simulink model "montecar"  (Simulink 4.00)
settings: Solver=VariableStepDiscrete  SolverMode=SingleTasking  StartTime=0.0  StopTime=10  FixedStep=1  MaxStep=1  RelTol=1e-3  AbsTol=1e-6
PreLoadFcn:
  | monteset
StopFcn:
  | monteplo
undefined symbols (not defined in the file or in its folder): fcost, invest, k, mshare, msize, pow, rate, ucost, uprice
CloseFcn:
  | close(findobj('name','Business Model Graph'))
settings Model: RequirementInfo=9  Creator=pseca  LastModifiedBy=eyarrow  SaveTime=off  SaveOutput=off  LimitDataPoints=off  RTWTemplateMakefile=grt_vc.tmf  BlockReductionOpt=off

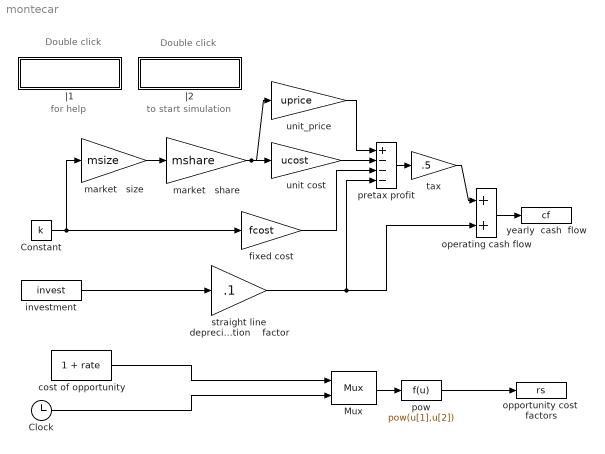
== system montecar ==
  note: Double click
  note: for help
  note: Double click
  note: to start simulation
  " straight line depreciation    factor" : Gain  Gain=.1  Multiplication=Element-wise(K.*u)  SaturateOnIntegerOverflow=on
  Clock : Clock
      settings: Decimation=10
  Constant : Constant  Value=k
  Mux : Mux  Inputs=2
      settings: DisplayOption=none
  "cost of opportunity " : Constant  Value=1 + rate
  fixed cost : Gain  Gain=fcost  Multiplication=Element-wise(K.*u)  SaturateOnIntegerOverflow=on
  investment : Constant  Value=invest
  market   share : Gain  Gain=mshare  Multiplication=Element-wise(K.*u)  SaturateOnIntegerOverflow=on
  market   size : Gain  Gain=msize  Multiplication=Element-wise(K.*u)  SaturateOnIntegerOverflow=on
  operating cash flow : Sum  Inputs=++  SaturateOnIntegerOverflow=on
  opportunity cost  factors : ToWorkspace  VariableName=rs  SampleTime=0  SaveFormat=Array
      settings: MaxDataPoints=10
  pow : Fcn  Expr=pow(u[1],u[2])
  pretax profit : Sum  Inputs=+---  SaturateOnIntegerOverflow=on
  tax : Gain  Gain=.5  Multiplication=Element-wise(K.*u)  SaturateOnIntegerOverflow=on
  unit cost : Gain  Gain=ucost  Multiplication=Element-wise(K.*u)  SaturateOnIntegerOverflow=on
  unit_price : Gain  Gain=uprice  Multiplication=Element-wise(K.*u)  SaturateOnIntegerOverflow=on
  yearly  cash  flow : ToWorkspace  VariableName=cf  SampleTime=0  SaveFormat=Array
      settings: MaxDataPoints=10
  |1 : Subsystem
      settings: OpenFcn=montehel  RTWFcnNameOpts=Auto  RTWFileNameOpts=Auto
      mask Display: disp('Help')
  |2 : Subsystem
      settings: OpenFcn=set_param(get_param(0,'currentsystem'),'simulationcommand','start')  RTWFcnNameOpts=Auto  RTWFileNameOpts=Auto
      mask Type: Start
      mask Help: Double click to start simulation
      mask Display: disp('Start')
  wires:
  unit cost/1 -> pretax profit/2
  pretax profit/1 -> tax/1
  unit_price/1 -> pretax profit/1
  investment/1 -> " straight line depreciation    factor"/1
  Clock/1 -> Mux/2
  Mux/1 -> pow/1
  "cost of opportunity "/1 -> Mux/1
  pow/1 -> opportunity cost  factors/1
  operating cash flow/1 -> yearly  cash  flow/1
  fixed cost/1 -> pretax profit/3
  market   size/1 -> market   share/1
  market   share/1 -> unit cost/1, unit_price/1
  tax/1 -> operating cash flow/1
  " straight line depreciation    factor"/1 -> operating cash flow/2, pretax profit/4
  Constant/1 -> fixed cost/1, market   size/1

== system montecar/|1 ==

== system montecar/|2 ==
